simulink model "impulse"  (R2020b)
settings: Solver=VariableStepAuto  StartTime=0.0  StopTime=10.0  RelTol=1e-3
settings Model: Creator=Ani  LastModifiedBy=Ani

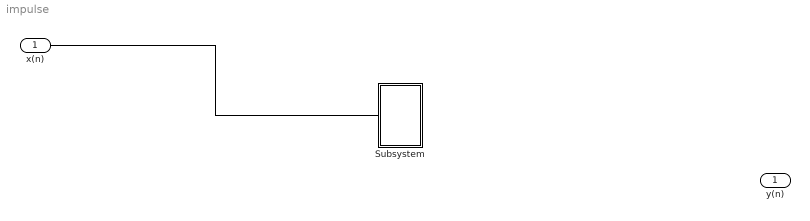
== system impulse ==
  x(n) : Inport  OutDataTypeStr=double  PortDimensions=1  SampleTime=[0,1]
  Subsystem : Subsystem
  y(n) : Outport  OutDataTypeStr=double  PortDimensions=1  SampleTime=[0,1]
  wires:
  x(n)/1 -> ?
  ? -> y(n)/1

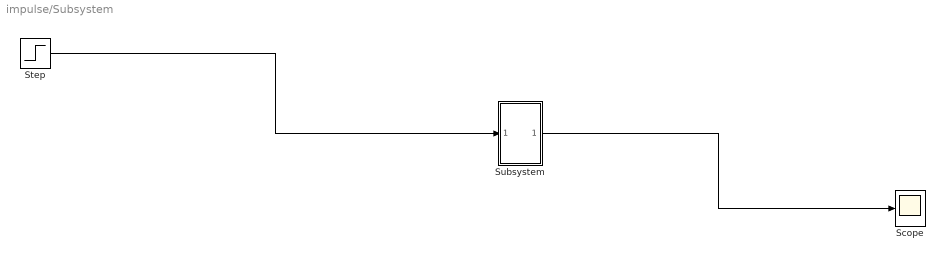
== system impulse/Subsystem ==
  Scope : Scope
  Step : Step  SampleTime=0
  Subsystem : Subsystem
  wires:
  Step/1 -> Subsystem/1(x(n))
  Subsystem/1(y(n)) -> Scope/1

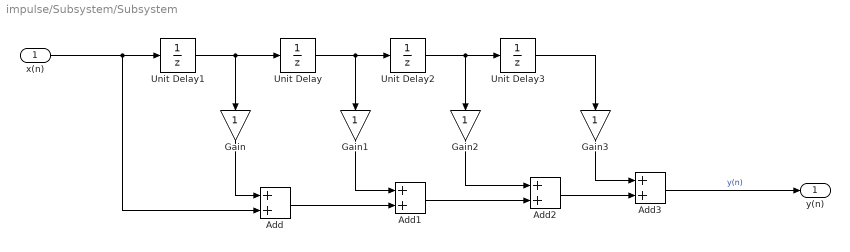
== system impulse/Subsystem/Subsystem ==
  x(n) : Inport  OutDataTypeStr=double  PortDimensions=1  SampleTime=[0,1]
  Add{,1..3} (4 alike) : Sum
  Gain{,1..3} (4 alike) : Gain
  Unit Delay{,1..3} (4 alike) : UnitDelay  SampleTime=-1  HasFrameUpgradeWarning=on
  y(n) : Outport  OutDataTypeStr=double  PortDimensions=1  SampleTime=[0,1]
  wires:
  Add3/1 -> y(n)/1  "y(n)"
  Add/1 -> Add1/2
  Unit Delay3/1 -> Gain3/1
  Unit Delay2/1 -> Unit Delay3/1, Gain2/1
  Gain2/1 -> Add2/1
  Unit Delay1/1 -> Unit Delay/1, Gain/1
  Gain/1 -> Add/1
  Unit Delay/1 -> Unit Delay2/1, Gain1/1
  Gain1/1 -> Add1/1
  Add1/1 -> Add2/2
  x(n)/1 -> Unit Delay1/1, Add/2
  Gain3/1 -> Add3/1
  Add2/1 -> Add3/2
